simulink model "ros2node_vis"  (R2024b)
settings: Solver=VariableStepAuto  StartTime=0.0  StopTime=10.0  RelTol=1e-3
settings Model: Creator=Alyssa  LastModifiedBy=Alyssa

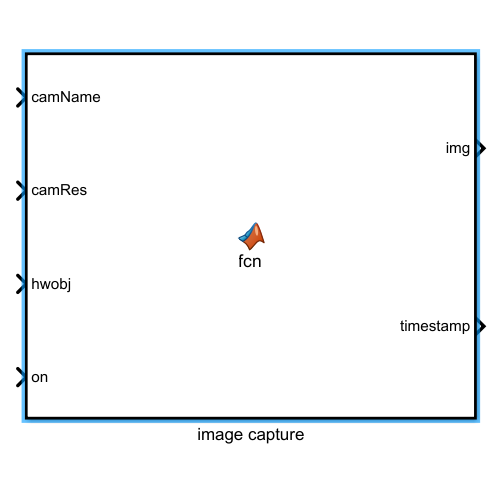
[thumbnail: Simulink's stored preview of the top-level diagram]
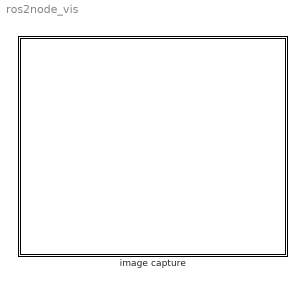
== system ros2node_vis ==
  image capture : MATLAB Function  TreatAsAtomicUnit=on

== matlab function ros2node_vis/image capture ==
function fcn()
 
nanoImgCapture();
